simulink model "Stepdown_cases"  (R2024b)
settings: Solver=VariableStepAuto  StartTime=0.0  StopTime=10.0  RelTol=1e-3
settings Model: Creator=Viral B Kalariya  LastModifiedBy=Viral B Kalariya

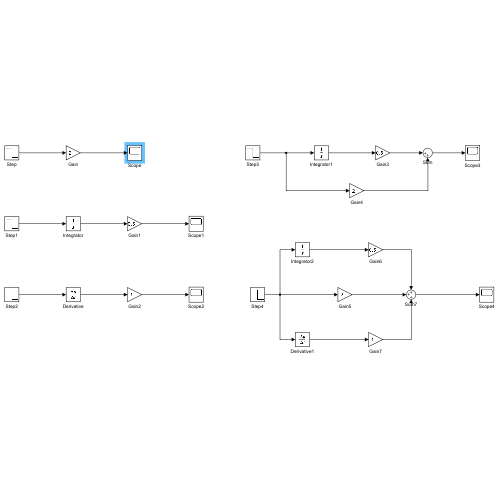
[thumbnail: Simulink's stored preview of the top-level diagram]
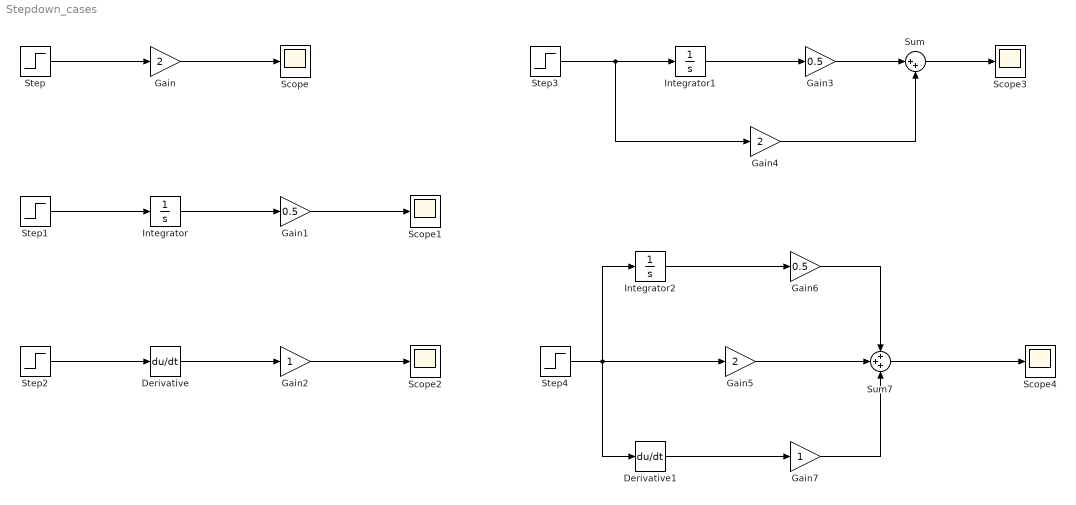
== system Stepdown_cases ==
  Derivative : Derivative
  Derivative1 : Derivative
  Gain : Gain  Gain=2
  Gain1 : Gain  Gain=0.5
  Gain2 : Gain
  Gain3 : Gain  Gain=0.5
  Gain4 : Gain  Gain=2
  Gain5 : Gain  Gain=2
  Gain6 : Gain  Gain=0.5
  Gain7 : Gain
  Integrator : Integrator
  Integrator1 : Integrator
  Integrator2 : Integrator
  Scope{,1..4} (5 alike) : Scope
  Step{,1..4} (5 alike) : Step  Time=2  Before=5  After=0  SampleTime=0
  Sum : Sum  Inputs=|++
  Sum7 : Sum  Inputs=+++
  wires:
  Step/1 -> Gain/1
  Gain/1 -> Scope/1
  Integrator/1 -> Gain1/1
  Step1/1 -> Integrator/1
  Gain1/1 -> Scope1/1
  Step2/1 -> Derivative/1
  Derivative/1 -> Gain2/1
  Gain2/1 -> Scope2/1
  Step3/1 -> Integrator1/1, Gain4/1
  Integrator1/1 -> Gain3/1
  Sum/1 -> Scope3/1
  Gain3/1 -> Sum/1
  Gain4/1 -> Sum/2
  Step4/1 -> Derivative1/1, Integrator2/1, Gain5/1
  Gain5/1 -> Sum7/2
  Sum7/1 -> Scope4/1
  Integrator2/1 -> Gain6/1
  Derivative1/1 -> Gain7/1
  Gain6/1 -> Sum7/1
  Gain7/1 -> Sum7/3
